simulink model "pv_system_monitoring"  (R2023a)
settings: Solver=VariableStepAuto  StartTime=0.0  StopTime=time(end)  RelTol=1e-3
settings Model: Creator=USER  LastModifiedBy=USER

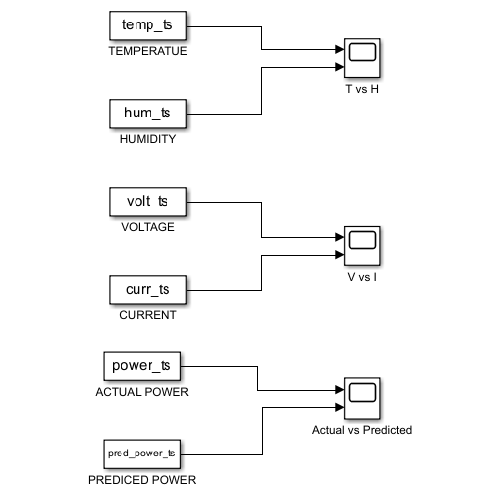
[thumbnail: Simulink's stored preview of the top-level diagram]
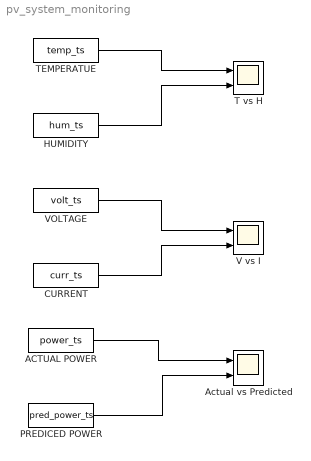
== system pv_system_monitoring ==
  ACTUAL POWER : FromWorkspace  VariableName=power_ts  SampleTime=-1
  Actual vs Predicted : Scope  NumInputPorts=2
  CURRENT : FromWorkspace  VariableName=curr_ts  SampleTime=-1
  "HUMIDITY " : FromWorkspace  VariableName=hum_ts  SampleTime=-1
  PREDICED POWER : FromWorkspace  VariableName=pred_power_ts  SampleTime=-1
  T vs H : Scope  NumInputPorts=2
  TEMPERATUE : FromWorkspace  VariableName=temp_ts  SampleTime=-1
  V vs I : Scope  NumInputPorts=2
  VOLTAGE : FromWorkspace  VariableName=volt_ts  SampleTime=-1
  wires:
  TEMPERATUE/1 -> T vs H/1
  "HUMIDITY "/1 -> T vs H/2
  VOLTAGE/1 -> V vs I/1
  CURRENT/1 -> V vs I/2
  ACTUAL POWER/1 -> Actual vs Predicted/1
  PREDICED POWER/1 -> Actual vs Predicted/2
